simulink model "optimalLQControl"  (R2015a)
settings: Solver=ode45  StartTime=0.0  StopTime=tijd  RelTol=1e-3
values from neighbouring files (symbols this model uses):
  A = [b1-d1-Y*a 0 0 ... (first row only)    [LQControl.m]    (also in LQControl_script.m; optimalLQControl_script.m = [-(beta1+c) 3*beta2)
  B = [1;0;0]    [LQControl.m]    (also in LQControl_script.m; optimalLQControl_script.m = [-1;0])
  C = [1 0 0 ... (first row only)    [LQControl.m]    (also in LQControl_script.m; optimalLQControl_script.m = [1 0)
  D = [0;0;0]    [LQControl.m]    (also in LQControl_script.m; optimalLQControl_script.m = [0;0])
  K1 = -k    [optimalLQControl_script.m]
  K2 = inv(R)*B'*(M+inv(A'-M*B*inv(R)*B')*M)    [optimalLQControl_script.m]
  n0 = 10    [optimalLQControl_script.m]
  U0 = 0    [optimalLQControl_script.m]
  X_sp = [10^4 10^3]    [optimalLQControl_script.m]
settings Model: Creator=Ward  LastModifiedBy=Ward

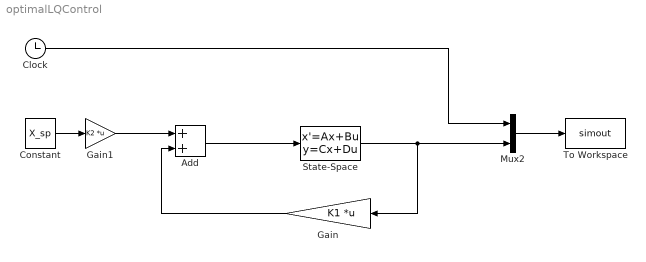
== system optimalLQControl ==
  Add : Sum
  Clock : Clock
  Constant : Constant  Value=X_sp
  Gain : Gain  Gain=K1  Multiplication=Matrix(K*u)
  Gain1 : Gain  Gain=K2  Multiplication=Matrix(K*u)
  Mux2 : Mux  Inputs=2
  State-Space : StateSpace  A=A  B=B  C=C  D=D  X0=[n0;U0]
  To Workspace : ToWorkspace  VariableName=simout  SampleTime=-1
  wires:
  State-Space/1 -> Gain/1, Mux2/2
  Clock/1 -> Mux2/1
  Mux2/1 -> To Workspace/1
  Constant/1 -> Gain1/1
  Gain1/1 -> Add/1
  Gain/1 -> Add/2
  Add/1 -> State-Space/1
